simulink model "sim_3dof_plane"  (R2016a)
settings: Solver=VariableStepAuto  StartTime=0.0  StopTime=40  RelTol=1e-3
settings Model: Creator=harith  LastModifiedBy=harith
settings GRTTargetCC: GeneratePreprocessorConditionals=Use local settings

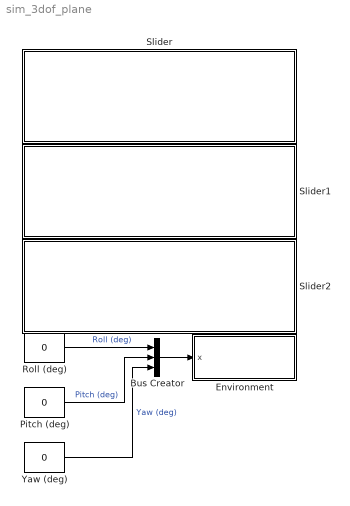
== system sim_3dof_plane ==
  Bus Creator : BusCreator  Inputs=3
  Environment : Subsystem
  Pitch (deg) : Constant  Value=0
  Roll (deg) : Constant  Value=0
  Slider : Subsystem  DialogController=hmiCreateDDGDialog  IsWebBlock=on  mask(MWDashboardBlock){webBlockId=49f42e52-404c-47e4-95dd-9776fa2b9152, webBlockType=slider, ShowInLibBrowser=on, ShowInitialText=on, HMISrcModelName=sim_3dof_plane}
      mask prompts: webBlockId "WebBlock Id"; webBlockType "WebBlock Type"; HMISrcModelName "Source Model"
      mask Help: helpview([docroot '/mapfiles/simulink.map'], 'hmi_slider')
      mask Display:
      | if strcmp(get_param(bdroot(gcb),'BlockDiagramType'), 'library')
      |     image([(matlabroot) '/toolbox/simulink/hmi/icons/Slider.png']);
      | end
  Slider1 : Subsystem  DialogController=hmiCreateDDGDialog  IsWebBlock=on  mask(MWDashboardBlock){webBlockId=1aa4d3d1-6060-4cd8-ae34-83414059d4d3, webBlockType=slider, ShowInLibBrowser=on, ShowInitialText=on, HMISrcModelName=sim_3dof_plane}
      mask prompts: webBlockId "WebBlock Id"; webBlockType "WebBlock Type"; HMISrcModelName "Source Model"
      mask Help: helpview([docroot '/mapfiles/simulink.map'], 'hmi_slider')
      mask Display:
      | if strcmp(get_param(bdroot(gcb),'BlockDiagramType'), 'library')
      |     image([(matlabroot) '/toolbox/simulink/hmi/icons/Slider.png']);
      | end
  Slider2 : Subsystem  DialogController=hmiCreateDDGDialog  IsWebBlock=on  mask(MWDashboardBlock){webBlockId=1c0d2ab2-9176-44ee-9c5b-bcbaa38d2a44, webBlockType=slider, ShowInLibBrowser=on, ShowInitialText=on, HMISrcModelName=sim_3dof_plane}
      mask prompts: webBlockId "WebBlock Id"; webBlockType "WebBlock Type"; HMISrcModelName "Source Model"
      mask Help: helpview([docroot '/mapfiles/simulink.map'], 'hmi_slider')
      mask Display:
      | if strcmp(get_param(bdroot(gcb),'BlockDiagramType'), 'library')
      |     image([(matlabroot) '/toolbox/simulink/hmi/icons/Slider.png']);
      | end
  Yaw (deg) : Constant  Value=0
  wires:
  Bus Creator/1 -> Environment/1(x)
  Roll (deg)/1 -> Bus Creator/1  "Roll (deg)"
  Pitch (deg)/1 -> Bus Creator/2  "Pitch (deg)"
  Yaw (deg)/1 -> Bus Creator/3  "Yaw (deg)"

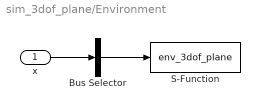
== system sim_3dof_plane/Environment ==
  x : Inport
  Bus Selector : BusSelector  OutputSignals=Roll (deg),Pitch (deg),Yaw (deg)  OutputAsBus=on
  S-Function : S-Function  FunctionName=env_3dof_plane  Parameters=[1 1],1,1  SFunctionDeploymentMode=off  EnableBusSupport=off
  wires:
  x/1 -> Bus Selector/1
  Bus Selector/1 -> S-Function/1

== system sim_3dof_plane/Slider ==

== system sim_3dof_plane/Slider1 ==

== system sim_3dof_plane/Slider2 ==
